simulink model "pendol_lqg"  (R2026a)
settings: Solver=FixedStepAuto  FixedStep=0.01
undefined symbols (not defined in the file): Akf, b, Bkf, c, Ckf, Dkf, g, I, kb, KK, kt, l, M, m, r, Rm
libraries: simulink x2
settings Model: Creator=jitendra  LastModifiedBy=berta
settings DataIOCC: ExternalInput=getinputstruct(op_trim1)  InitialState=getstatestruct(op_trim1)

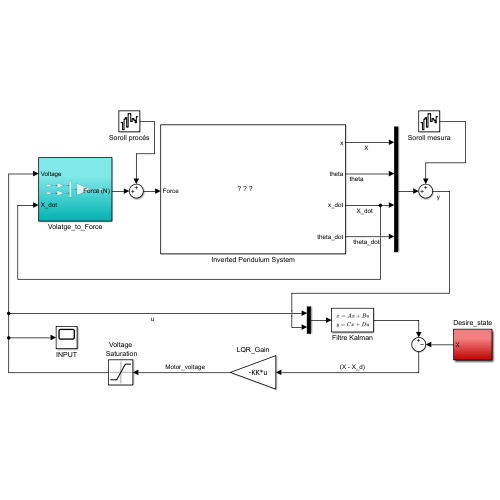
[thumbnail: Simulink's stored preview of the top-level diagram]
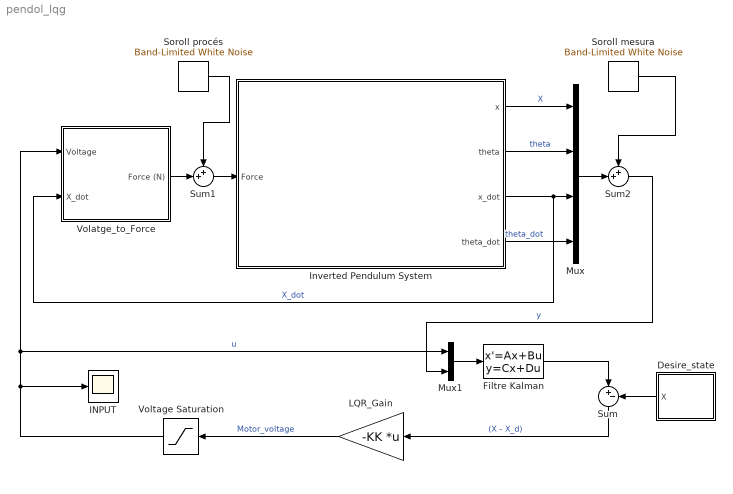
== system pendol_lqg ==
  Desire_state : Subsystem
  Filtre Kalman : StateSpace  A=Akf  B=Bkf  C=Ckf  D=Dkf  InitialCondition=0
  INPUT : Scope
      settings: ActiveDisplayYMinimum=-12  ActiveDisplayYMaximum=12
  Inverted Pendulum System : Subsystem
      mask Display: image('pendol.png');
  LQR_Gain : Gain  Gain=-KK  Multiplication=Matrix(K*u)
  Mux : Mux
  Mux1 : Mux  Inputs=[1; 4]
  Soroll mesura : simulink/Sources/Band-Limited White Noise  Cov=[0.0001 0.0001 0.0001 0.0001]  Ts=0.1  seed=[23341]
  Soroll procés : simulink/Sources/Band-Limited White Noise  Cov=0.0001  Ts=0.1  seed=[23341]
  Sum : Sum  Inputs=|+-
  Sum1 : Sum  Inputs=++|
  Sum2 : Sum  Inputs=++|
  Volatge_to_Force : Subsystem
  Voltage Saturation : Saturate  UpperLimit=10  LowerLimit=-10
  wires:
  Inverted Pendulum System/3(x_dot) -> Volatge_to_Force/2(X_dot), Mux/3  "X_dot"
  Inverted Pendulum System/1(x) -> Mux/1  "X"
  Inverted Pendulum System/4(theta_dot) -> Mux/4  "theta_dot"
  LQR_Gain/1 -> Voltage Saturation/1  "Motor_voltage"
  Desire_state/1(X) -> Sum/2
  Sum/1 -> LQR_Gain/1  "(X - X_d)"
  Voltage Saturation/1 -> Volatge_to_Force/1(Voltage), Mux1/1, INPUT/1  "u"
  Volatge_to_Force/1(Force (N)) -> Sum1/2
  Soroll procés/1 -> Sum1/1
  Sum1/1 -> Inverted Pendulum System/1(Force)
  Mux/1 -> Sum2/2
  Soroll mesura/1 -> Sum2/1
  Mux1/1 -> Filtre Kalman/1
  Filtre Kalman/1 -> Sum/1
  Sum2/1 -> Mux1/2  "y"
  Inverted Pendulum System/2(theta) -> Mux/2  "theta"

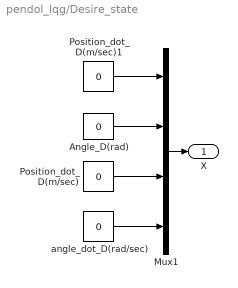
== system pendol_lqg/Desire_state ==
  Angle_D(rad) : Constant  Value=0
  Mux1 : Mux
  Position_dot_D(m/sec) : Constant  Value=0
  Position_dot_D(m/sec)1 : Constant  Value=0
  angle_dot_D(rad/sec) : Constant  Value=0
  X : Outport  VectorParamsAs1DForOutWhenUnconnected=off
  wires:
  Mux1/1 -> X/1
  Position_dot_D(m/sec)/1 -> Mux1/3
  angle_dot_D(rad/sec)/1 -> Mux1/4
  Angle_D(rad)/1 -> Mux1/2
  Position_dot_D(m/sec)1/1 -> Mux1/1

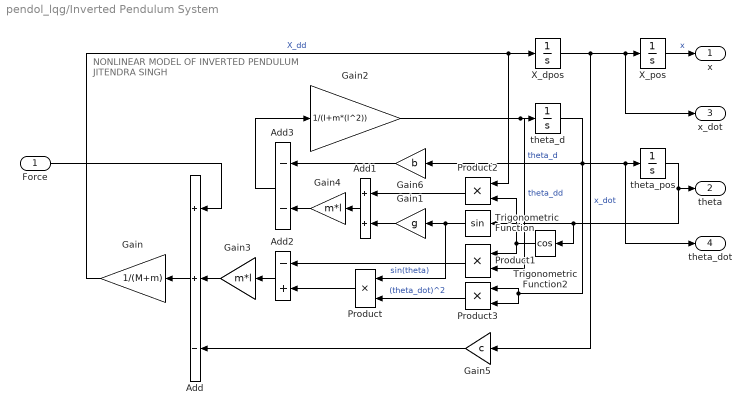
== system pendol_lqg/Inverted Pendulum System ==
  note: NONLINEAR MODEL OF
      | INVERTED PENDULUM
      | JITENDRA SINGH
  Force : Inport
  Add : Sum  Inputs=++-
  Add1 : Sum
  Add2 : Sum  Inputs=-+
  Add3 : Sum  Inputs=--
  Gain : Gain  Gain=1/(M+m)
  Gain1 : Gain  Gain=g
  Gain2 : Gain  Gain=1/(I+m*(l^2))
  Gain3 : Gain  Gain=m*l
  Gain4 : Gain  Gain=m*l
  Gain5 : Gain  Gain=c
  Gain6 : Gain  Gain=b
  Product{,1..3} (4 alike) : Product
  Trigonometric Function : Trigonometry
  Trigonometric Function2 : Trigonometry  Operator=cos
  X_dpos : Integrator
  X_pos : Integrator  InitialCondition=0.2
  theta_d : Integrator
  theta_pos : Integrator  InitialCondition=pi*(1-0.1)
  x : Outport  VectorParamsAs1DForOutWhenUnconnected=off
  theta : Outport  Port=2  VectorParamsAs1DForOutWhenUnconnected=off
  x_dot : Outport  Port=3  VectorParamsAs1DForOutWhenUnconnected=off
  theta_dot : Outport  Port=4  VectorParamsAs1DForOutWhenUnconnected=off
  wires:
  Gain5/1 -> Add/3
  Add2/1 -> Gain3/1
  Add3/1 -> Gain2/1
  Trigonometric Function2/1 -> Product2/2, Product1/1
  Trigonometric Function/1 -> Product/1, Gain1/1  "sin(theta)"
  Gain3/1 -> Add/2
  theta_d/1 -> Product3/2, Product3/1, Gain6/1, theta_dot/1, theta_pos/1  "theta_d"
  Product2/1 -> Add1/1
  Product/1 -> Add2/2
  Gain4/1 -> Add3/2
  Product3/1 -> Product/2  "(theta_dot)^2"
  X_pos/1 -> x/1  "x"
  Product1/1 -> Add2/1
  Gain/1 -> X_dpos/1, Product2/1  "X_dd"
  Add/1 -> Gain/1
  Gain2/1 -> Product1/2, theta_d/1  "theta_dd"
  Gain6/1 -> Add3/1
  theta_pos/1 -> Trigonometric Function2/1, Trigonometric Function/1, theta/1
  Force/1 -> Add/1
  Gain1/1 -> Add1/2
  X_dpos/1 -> x_dot/1, X_pos/1, Gain5/1  "x_dot"
  Add1/1 -> Gain4/1

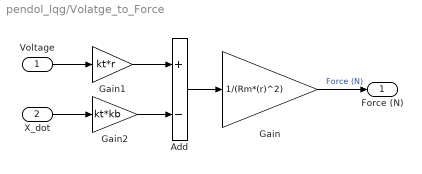
== system pendol_lqg/Volatge_to_Force ==
  Voltage : Inport
  X_dot : Inport  Port=2
  Add : Sum  Inputs=+-
  Gain : Gain  Gain=1/(Rm*(r)^2)
  Gain1 : Gain  Gain=kt*r
  Gain2 : Gain  Gain=kt*kb
  Force (N) : Outport  VectorParamsAs1DForOutWhenUnconnected=off
  wires:
  Gain1/1 -> Add/1
  Gain2/1 -> Add/2
  Voltage/1 -> Gain1/1
  Gain/1 -> Force (N)/1  "Force (N)"
  X_dot/1 -> Gain2/1
  Add/1 -> Gain/1
